simulink model "controllREAL_FINAL1"  (R2018a)
settings: Solver=VariableStepAuto  StartTime=0.0  StopTime=600  FixedStep=0.05  RelTol=1e-3
values from neighbouring files (symbols this model uses):
  C1 = [1 0]    [Lab1.m]
  C2 = [0 1]    [Lab1.m]
  h = 5:1:15    [Lab1.m]
  hV = [1.826, 2.539, 3.452, 4.18, 4.99, 5.762, 6.665, 7.36, 8.193, 8.93, 9.66]    [Lab1.m]
  K = K'    [Lab1.m]
  v = 1:1:10    [Lab1.m]
  vt = [21.18, 26.66 30.97, 34.28, 37.92, 39.73, 42.53, 45.45, 46.49, 47.67]    [Lab1.m]
undefined symbols (not defined in the file or in its folder): Ak, Bk, Ck, National_Instruments, PCI, sigbuilder_block
libraries: sldrtlib x2
settings Model: Creator=Scott  LastModifiedBy=oscbck-5
settings SolverCC: AlgebraicLoopSolver=LineSearch

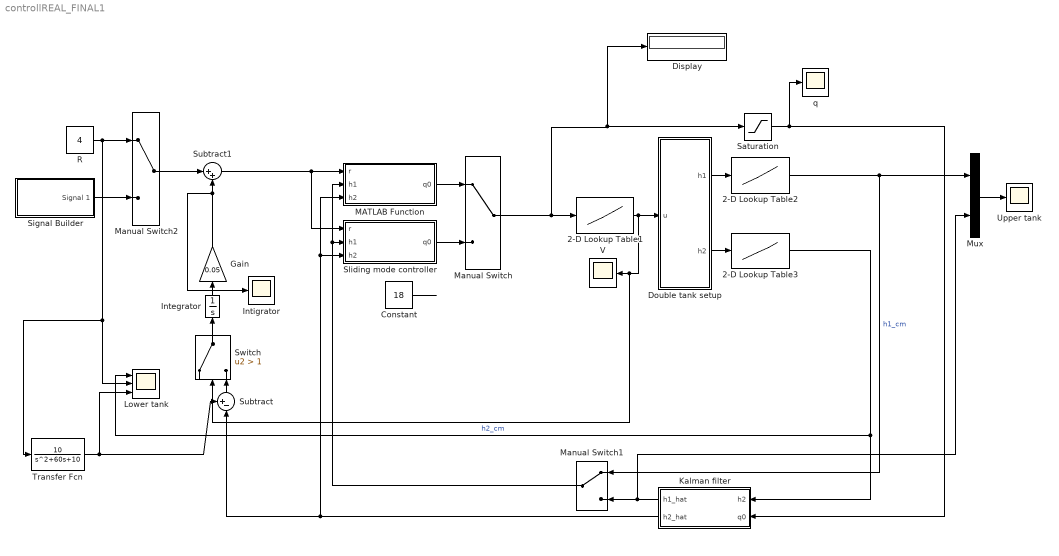
== system controllREAL_FINAL1 ==
  2-D Lookup Table1 : Lookup_n-D  NumberOfTableDimensions=1  BreakpointsForDimension1=x  BreakpointsForDimension2=[1:3]  Table=y  RndMeth=Simplest  InputSameDT=on  mask{x=vt, y=v}
      mask prompts: x "Values on x-axis"; y "Values on y-axis"
  2-D Lookup Table2 : Lookup_n-D  NumberOfTableDimensions=1  BreakpointsForDimension1=x  BreakpointsForDimension2=[1:3]  Table=y  RndMeth=Simplest  InputSameDT=on  mask{x=hV, y=h}
      mask prompts: x "Values on x-axis"; y "Values on y-axis"
  2-D Lookup Table3 : Lookup_n-D  NumberOfTableDimensions=1  BreakpointsForDimension1=x  BreakpointsForDimension2=[1:3]  Table=y  RndMeth=Simplest  InputSameDT=on  mask{x=hV, y=h}
      mask prompts: x "Values on x-axis"; y "Values on y-axis"
  Constant : Constant  Value=18
  Display : Display
  Double tank setup : Subsystem  AncestorBlock=R0002E_lib/Double tank setup  StopFcn=|  mask(Realtime interface for the tank process){ts=0.05, h1_ch=0, h2_ch=1, u_ch=0}
      | chn =get_param(gcb,'u_ch');                          
      | s = daq.createSession('ni');                         
      | channel = ['ao',chn];                                
      | s.addAnalogOutputChannel('Dev1', channel, 'Voltage');
      | x = zeros(5,1);                                      
      | s.queueOutputData(x);                                
      | lh = s.addlistener('DataRequired', ...               
      | @(src,event) src.queueOutputData(x));                
      | s.startBackground();                                 
      | s.wait();                                            
      | s.stop();                                            
      | delete(lh);                                          
      | clear chn;                                           
      | clear s;                                             
      | clear channel;                                       
      | clear lh;                                            
      | clear x;
      mask prompts: ts "Sample time"; h1_ch "A/D Channel for upper tank"; h2_ch "A/D Channel for lower tank"; u_ch "D/A Channel for pump"
      mask help:
      | This block represents the physical interface from the computer to the tank process.
      |
      | The input u is the voltage that is provided for the pump, the output h1 is the measured level in the upper tank in [V] and the output h2 is the
      | measured level in the lower tank in [V].
      |
      | You need to provide the sample rate at which the voltage to the pump is updated and the level measurements are sampled. The sample rate should not be less than 0.02 seconds.
      mask Display:
      | x=363;
      | y=381;
      | image(imread('tank_icon.jpg'));
      | text(250/x,309/y,'Sensor');
      | text(260/x,169/y,'Sensor');
      | text(335/x,289/y,'A');
      | text(351/x,283/y,'D');
      | text(335/x,100/y,'A');
      | text(351/x,95/y,'D');
      | text(22/x,187/y,'A');
      | text(5/x,195/y,'D');
      | text(225/x,278/y,'h_1','texmode','on');
      | text(225/x,146/y,'h_2','texmode','on');
      | text(300/x,270/y,sprintf('AI-%d',h1_ch));
      | text(300/x,80/y,sprintf('AI-%d',h2_ch));
      | text(40/x,173/y,sprintf('AO-%d',u_ch));
  Gain : Gain  Gain=0.05
  Integrator : Integrator
  "Intigrator " : Scope
  Kalman filter : Subsystem
  Lower tank : Scope  NumInputPorts=3
  MATLAB Function : MATLAB Function  TreatAsAtomicUnit=on
  Manual Switch : ManualSwitch
  Manual Switch1 : ManualSwitch
  Manual Switch2 : ManualSwitch
  Mux : Mux  Inputs=2
  R : Constant  Value=4
  Saturation : Saturate  UpperLimit=47  LowerLimit=0
  Signal Builder : Subsystem  Tag=STV Subsys  LoadFcn=sigbuilder_block('load');  StartFcn=sigbuilder_block('start');  StopFcn=sigbuilder_block('stop');  ClipboardFcn=sigbuilder_block('clipboard');  mask(Sigbuilder block){tuvar=[0:10]}
      mask help: Simulink:masks:SigbuilderBlock_MD
      mask init:
      | if ~strcmp(get_param(bdroot(gcbh),'SimulationStatus'),'stopped') tuvar = sigbuilder_block('maskInit'); end
      settings: CopyFcn=sigbuilder_block('copy');  DeleteFcn=sigbuilder_block('delete');  ModelCloseFcn=sigbuilder_block('modelClose');  PreSaveFcn=sigbuilder_block('preSave');  PauseFcn=sigbuilder_block('pause');  ContinueFcn=sigbuilder_block('continue');  NameChangeFcn=sigbuilder_block('namechange');  OpenFcn=sigbuilder_block('open',[643.5 95.25 483.75 400.5 ]);  CloseFcn=sigbuilder_block('close');
      mask Display: plot(0, 0, 100, 100,[2, 2, 32, 32, 2], [68, 8, 8, 68, 68],[32, 2], [38, 38], [32, 19, 2],[53, 60, 44], [32, 17, 17, 2],[16, 16, 31, 31]);txt = getActiveGroup(gcbh);text(2, 100, txt,'verticalAlignment', 'top');
  Sliding mode controller : MATLAB Function  TreatAsAtomicUnit=on
  Subtract : Sum  Inputs=+-|
  Subtract1 : Sum  Inputs=|++
  Switch : Switch  Criteria=u2 > Threshold  Threshold=1
  Transfer Fcn : TransferFcn  Numerator=[10]  Denominator=[1 60 10]
  Upper tank : Scope
  V : Scope
  q : Scope
  wires:
  2-D Lookup Table2/1 -> Mux/1, Manual Switch1/1  "h1_cm"
  2-D Lookup Table3/1 -> Kalman filter/1("h2 "), Lower tank/1  "h2_cm"
  MATLAB Function/1(q0) -> Manual Switch/1
  Signal Builder/1(Signal 1) -> Manual Switch2/2
  Kalman filter/2("h2_hat ") -> MATLAB Function/3(h2), Sliding mode controller/3(h2), Subtract/2
  Kalman filter/1(h1_hat) -> Mux/2, Manual Switch1/2
  Mux/1 -> Upper tank/1
  Manual Switch/1 -> Saturation/1, Display/1, 2-D Lookup Table1/1
  Sliding mode controller/1(q0) -> Manual Switch/2
  Manual Switch1/1 -> MATLAB Function/2(h1), Sliding mode controller/2(h1)
  R/1 -> Transfer Fcn/1, Lower tank/2, Manual Switch2/1
  Double tank setup/1(h1) -> 2-D Lookup Table2/1
  Double tank setup/2(h2) -> 2-D Lookup Table3/1
  Saturation/1 -> Kalman filter/2(q0), q/1
  Constant/1 -> ?
  Transfer Fcn/1 -> Subtract/1, Lower tank/3
  Integrator/1 -> Gain/1
  Switch/1 -> Integrator/1
  Manual Switch2/1 -> Subtract1/1
  Subtract1/1 -> MATLAB Function/1(r), Sliding mode controller/1(r)
  Subtract/1 -> Switch/3
  Gain/1 -> "Intigrator "/1, Subtract1/2
  2-D Lookup Table1/1 -> Switch/2, V/1, Double tank setup/1(u)

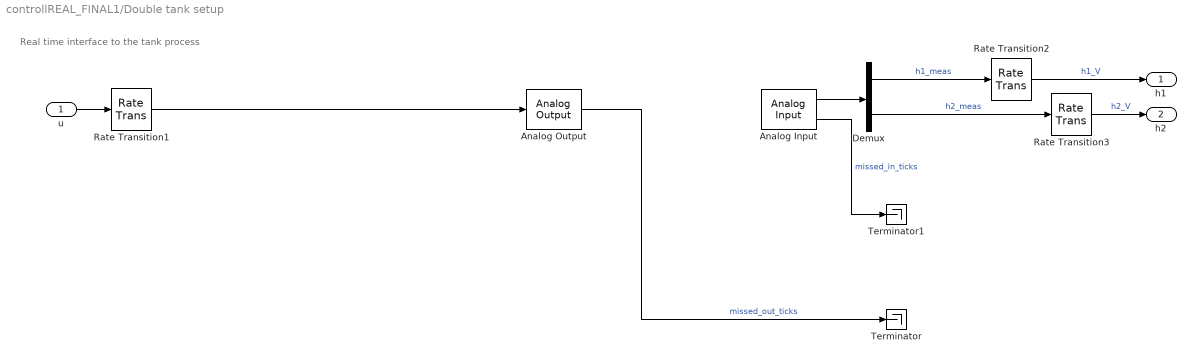
== system controllREAL_FINAL1/Double tank setup ==
  note: Real time interface to the tank process
  u : Inport
  Analog Input : sldrtlib/Analog Input  SampleTime=ts  MaxMissedTicks=500000000  ShowMissedTicks=on  YieldWhenWaiting=off  DrvName=National_Instruments/PCI-6024E  DrvAddress=4294967295  DrvOptions=[0 0 0 0 0 0]  Channels=[h1_ch+1,h2_ch+1]  RangeMode=1  VoltRange=1  DataType=1
      settings: AttributesFormatString=National Instruments\nPCI-6024E [auto]  SourceProductName=Simulink Desktop Real-Time
  Analog Output : sldrtlib/Analog Output  SampleTime=ts  MaxMissedTicks=500000000  ShowMissedTicks=on  YieldWhenWaiting=off  DrvName=National_Instruments/PCI-6024E  DrvAddress=4294967295  DrvOptions=[0 0 0 0 0 0]  Channels=u_ch+1  RangeMode=1  VoltRange=1  InitialValue=0  FinalValue=0
      settings: AttributesFormatString=National Instruments\nPCI-6024E [auto]  SourceProductName=Simulink Desktop Real-Time
  Demux : Demux  Outputs=2
  Rate Transition1 : RateTransition  OutPortSampleTime=ts
  Rate Transition2 : RateTransition
  Rate Transition3 : RateTransition
  Terminator : Terminator
  Terminator1 : Terminator
  h1 : Outport
  h2 : Outport  Port=2
  wires:
  Rate Transition1/1 -> Analog Output/1
  Rate Transition3/1 -> h2/1  "h2_V"
  Rate Transition2/1 -> h1/1  "h1_V"
  Analog Input/2 -> Terminator1/1  "missed_in_ticks"
  Demux/2 -> Rate Transition3/1  "h2_meas"
  Demux/1 -> Rate Transition2/1  "h1_meas"
  Analog Input/1 -> Demux/1
  Analog Output/1 -> Terminator/1  "missed_out_ticks"
  u/1 -> Rate Transition1/1

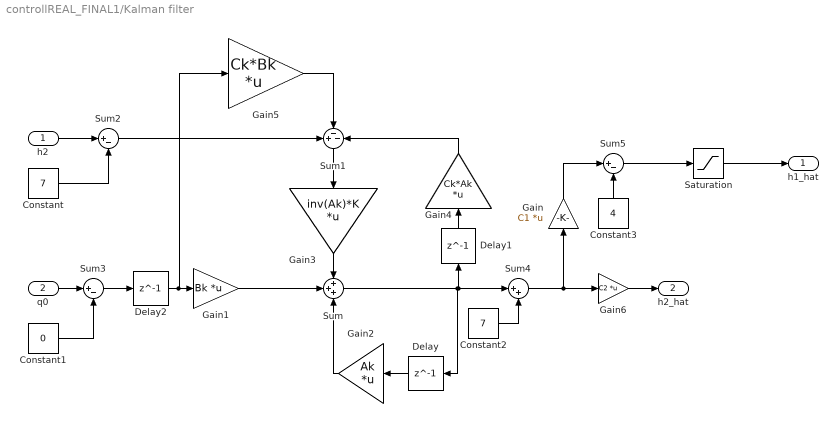
== system controllREAL_FINAL1/Kalman filter ==
  "h2 " : Inport
  q0 : Inport  Port=2
  Constant : Constant  Value=7
  Constant1 : Constant  Value=0
  Constant2 : Constant  Value=7
  Constant3 : Constant  Value=4
  Delay : Delay  DelayLength=1  InitialCondition=0  SampleTime=0.05
  Delay1 : Delay  DelayLength=1  InitialCondition=0  SampleTime=0.05
  Delay2 : Delay  DelayLength=1  InitialCondition=0  SampleTime=0.05
  Gain : Gain  Gain=C1  Multiplication=Matrix(K*u)
  Gain1 : Gain  Gain=Bk  Multiplication=Matrix(K*u)
  Gain2 : Gain  Gain=Ak  Multiplication=Matrix(K*u)
  Gain3 : Gain  Gain=inv(Ak)*K  Multiplication=Matrix(K*u)
  Gain4 : Gain  Gain=Ck*Ak  Multiplication=Matrix(K*u)
  Gain5 : Gain  Gain=Ck*Bk  Multiplication=Matrix(K*u)
  Gain6 : Gain  Gain=C2  Multiplication=Matrix(K*u)
  Saturation : Saturate  UpperLimit=15  LowerLimit=0
  Sum : Sum  Inputs=+++
  Sum1 : Sum  Inputs=+--
  Sum2 : Sum  Inputs=|+-
  Sum3 : Sum  Inputs=|+-
  Sum4 : Sum  Inputs=|++
  Sum5 : Sum  Inputs=|+-
  h1_hat : Outport
  "h2_hat " : Outport  Port=2
  wires:
  Gain5/1 -> Sum1/2
  Gain3/1 -> Sum/1
  Sum/1 -> Sum4/1, Delay1/1, Delay/1
  Delay2/1 -> Gain5/1, Gain1/1
  Gain4/1 -> Sum1/3
  Delay1/1 -> Gain4/1
  Gain1/1 -> Sum/2
  Sum1/1 -> Gain3/1
  Delay/1 -> Gain2/1
  Gain2/1 -> Sum/3
  "h2 "/1 -> Sum2/1
  Sum2/1 -> Sum1/1
  Constant/1 -> Sum2/2
  q0/1 -> Sum3/1
  Sum3/1 -> Delay2/1
  Constant1/1 -> Sum3/2
  Sum4/1 -> Gain/1, Gain6/1
  Constant2/1 -> Sum4/2
  Gain/1 -> Sum5/1
  Gain6/1 -> "h2_hat "/1
  Constant3/1 -> Sum5/2
  Sum5/1 -> Saturation/1
  Saturation/1 -> h1_hat/1

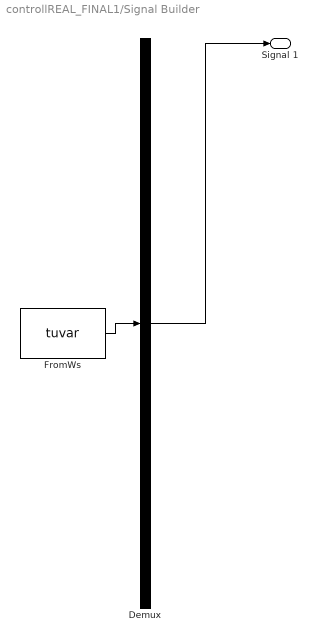
== system controllREAL_FINAL1/Signal Builder ==
  Demux : Demux  Tag=STV Demux  Outputs=1
  FromWs : FromWorkspace  Tag=STV FromWs  VariableName=tuvar  SampleTime=0
      SigBuilderData=|
      | common.afterFinalStr = 'Extrapolate'
      | common.sampleTime = 0
      | dataSet.timeRange = [0 60]
      | dataSet.name = 'Group 1'
      | sbobj.Groups.Name = 'Group 1'
      | sbobj.Groups.Signals.Name = 'Signal 1'
      | sbobj.Groups.Signals.XData = [0 4 20 40 58 60]
      | sbobj.Groups.Signals.YData = [0 0 7 1 5 5]
      | sbobj.Groups.TimeRange = [0 60]
  Signal 1 : Outport  Tag=STV Outport
  wires:
  Demux/1 -> Signal 1/1
  FromWs/1 -> Demux/1

== matlab function controllREAL_FINAL1/MATLAB Function ==
  data: r input; q0 output; h1 input; h2 input
function q0 = fcn(r,h1,h2)
%const
g = 981;
A=33;
a=0.17;
h0=3.2;

L=[10 60];
Lr=L(1);
ep=[h2
    a/+A*(sqrt(2*g*(h1+h0))-sqrt(2*g*(h2+h0)))];

alfa=2*sqrt(g*(h1+h0))*A/(a*g*sqrt(2));
beta=a^2*(g*(1/A^2-1/A)-g*sqrt(g*(h1+h0))/(sqrt(g*(h2+h0))*A^2));

q0=alfa*(-beta+Lr*r-L*ep);

end

== matlab function controllREAL_FINAL1/Sliding mode controller ==
  data: r input; q0 output; h1 input; h2 input
function q0 = fcn(r,h1,h2)
%const
g = 981;
A=33;
a=0.17;
h0=3.2;

%Controller cons
my=10;
ep=0.5;
P=[1 3];

%Controller vectors
Z=[h2-r
   a/A*(sqrt(2*g*(h1+h0))-sqrt(2*g*(h2+h0)))];
F=[a/A*(sqrt(2*g*(h1+h0))-sqrt(2*g*(h2+h0)))
   a^2*(g*(1/A^2-1/A)-g*sqrt(g*(h1+h0))/(A^2*sqrt(h2+h0)))];
G=[0
   a*g*sqrt(2)/(2*A*sqrt(g*(h1+h0)))];

sigma=P*Z;
if abs(sigma)<ep
   sat=sigma /ep;
else
   sat=sign(sigma);
end

q0=-P*F/(P*G)-my/(P*G)*sat;

if h1>15
    q0=10;
end
end
